simulink model "c8mexp2s"  (R2022a)
settings: Solver=VariableStepAuto  StartTime=0.0  StopTime=1  FixedStep=0.001  RelTol=1e-11  EnableMultiTasking=on
PreLoadFcn:
  | ww=[1e-4 1e4]; N=9;
libraries: cstblocks x2
settings Model: Creator=toshiba  LastModifiedBy=xuedi
settings SolverCC: AlgebraicLoopSolver=TrustRegion
settings DataIOCC: LimitDataPoints=on  MaxDataPoints=10000  SaveFormat=Array  SignalLoggingSaveFormat=ModelDataLogs  ReturnWorkspaceOutputs=off
settings OptimizationCC: ExpressionDepthLimit=2147483647  LifeSpan=inf
settings DebuggingCC: UnderspecifiedInitializationDetection=Classic  MergeDetectMultiDrivingBlocksExec=none  SolverPrmCheckMsg=warning  FcnCallInpInsideContextMsg=warning  UnconnectedInputMsg=warning  UnconnectedOutputMsg=warning  UnconnectedLineMsg=warning  AllowSymbolicDim=off  StateNameClashWarn=warning  SFUnexpectedBacktrackingDiag=warning  SFNoUnconditionalDefaultTransitionDiag=warning  SFExecutionAtInitializationDiag=none  SFMachineParentedDataDiag=warning  ArithmeticOperatorsInVariantConditions=warning
settings HardwareCC: ProdBitPerPointer=32  ProdBitPerSizeT=32  ProdBitPerPtrDiffT=32  ProdLargestAtomicFloat=None  ProdIntDivRoundTo=Undefined  ProdEndianess=Unspecified  ProdWordSize=32  ProdHWDeviceType=32-bit Generic
settings ModelReferenceCC: PropagateSignalLabelsOutOfModel=off
settings SFSimCC: SimUseLocalCustomCode=off  CustomCodeUndefinedFunction=UseInterfaceOnly
settings RTWCC: RTWUseLocalCustomCode=off  DLArmComputeVersion=19.05
settings CodeAppCC: StateflowObjectComments=on
settings GRTTargetCC: TargetLangStandard=C89/C90 (ANSI)  CombineOutputUpdateFcns=off  GRTInterface=on
settings ConfigComp: CovMetricSettings=dw  CovSaveCumulativeToWorkspaceVar=on  CovSaveSingleToWorkspaceVar=on  CovExternalEMLEnable=off

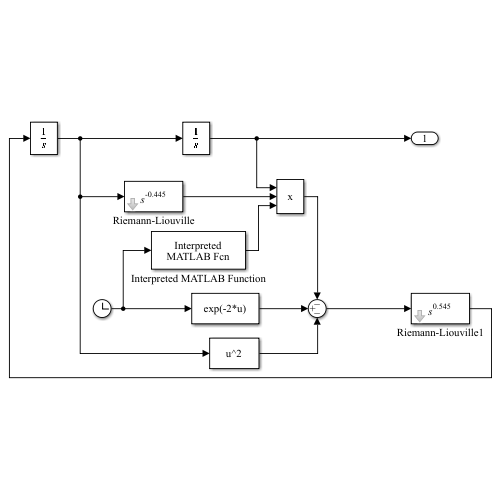
[thumbnail: Simulink's stored preview of the top-level diagram]
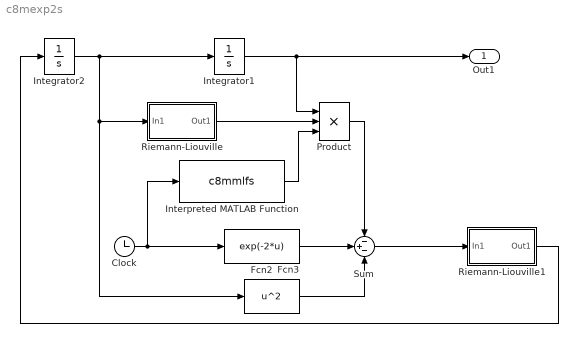
== system c8mexp2s ==
  Clock : Clock
  Fcn2 : Fcn  Expr=exp(-2*u)
  Fcn3 : Fcn  Expr=u^2
  Integrator1 : Integrator  InitialCondition=1
  Integrator2 : Integrator  InitialCondition=-1
  Interpreted MATLAB Function : MATLABFcn  MATLABFcn=c8mmlfs
  Product : Product  Inputs=***  RndMeth=Zero
  Riemann-Liouville : Subsystem  mask{gam=-0.445, ww=ww, n=N, kF1=off, kF=Oustaloup filter}
      mask prompts: gam "Derivative order gamma"; ww "Frequency range [wb,wh]"; n "Apprixmation order"; kF1 "Is a low-pass filter required?"; kF "Filter type"
      mask init:
      | wb=ww(1); wh=ww(2); 
      |    if isnumeric(gam), str=['{\its}^{' num2str(gam) '}']; 
      |    else, str='{\its}^{\gamma}'; end
      |    switch kF
      |       case 1, G=ousta_fod(gam,n,wb,wh);
      |       case 2, G=new_fod(gam,n,wb,wh); 
      |       case 3, G=matsuda_fod(gam,n,wb,wh); 
      |       case 4, G=srid_fod(gam,0.01,n);
      |    end
      |    T=1e-6/wh; if kF1==1, G=G*tf(1,[T 1]); end
      mask TypeOptions kF: Oustaloup filter | Modified Oustaloup filter | Matsuda-Fujii filter | Discrete step invariant filter
      mask Display: disp(str,'texmode','on')
  Riemann-Liouville1 : Subsystem  mask{gam=0.545, ww=ww, n=N, kF1=off, kF=Oustaloup filter}
      mask prompts: gam "Derivative order gamma"; ww "Frequency range [wb,wh]"; n "Apprixmation order"; kF1 "Is a low-pass filter required?"; kF "Filter type"
      mask init: same as c8mexp2s/Riemann-Liouville
      mask TypeOptions kF: Oustaloup filter | Modified Oustaloup filter | Matsuda-Fujii filter | Discrete step invariant filter
      mask Display: disp(str,'texmode','on')
  Sum : Sum  Inputs=-+-
  Out1 : Outport
  wires:
  Integrator1/1 -> Out1/1, Product/1
  Clock/1 -> Fcn2/1, Interpreted MATLAB Function/1
  Fcn2/1 -> Sum/2
  Fcn3/1 -> Sum/3
  Interpreted MATLAB Function/1 -> Product/3
  Product/1 -> Sum/1
  Integrator2/1 -> Riemann-Liouville/1(In1), Fcn3/1, Integrator1/1
  Sum/1 -> Riemann-Liouville1/1(In1)
  Riemann-Liouville/1(Out1) -> Product/2
  Riemann-Liouville1/1(Out1) -> Integrator2/1

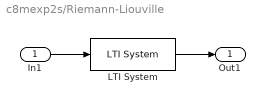
== system c8mexp2s/Riemann-Liouville ==
  In1 : Inport
  LTI System : cstblocks/LTI System  sys=G  IC=[]
  Out1 : Outport
  wires:
  In1/1 -> LTI System/1
  LTI System/1 -> Out1/1

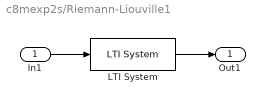
== system c8mexp2s/Riemann-Liouville1 ==
  In1 : Inport
  LTI System : cstblocks/LTI System  sys=G  IC=[]
  Out1 : Outport
  wires:
  LTI System/1 -> Out1/1
  In1/1 -> LTI System/1
